simulink model "HardwareM2Eq5"  (R2015a)
settings: configuration reference "SIMULATION_CONFIGURATION" (kept outside this file)
settings Model: DSRTSU_INTERNAL_RTI_VER=400  DSRTSU_INTERNAL_RTI_TYPE=rti1103  SimulationMode=accelerator  CovSFcnEnable=off  Creator=DIT  LastModifiedBy=moritz
settings ConfigSetRef: SourceLocation=Base Workspace

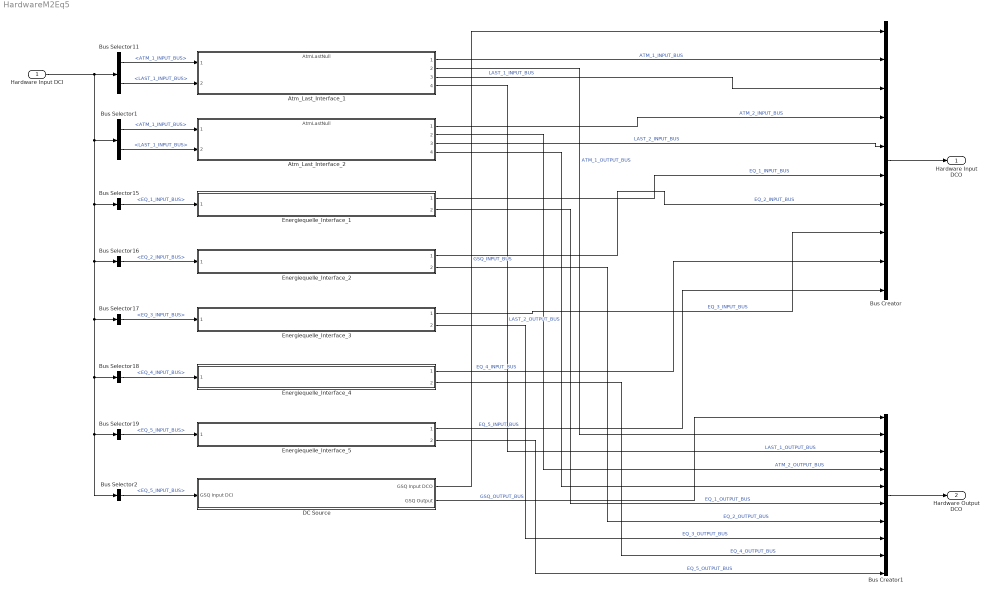
== system HardwareM2Eq5 ==
  Hardware Input DCI : Inport  OutDataTypeStr=Bus: HARDWARE_INPUT_BUS  BusOutputAsStruct=on
  Atm_Last_Interface_1 : ModelReference  ModelNameDialog=AtmLastNull  Variant=on  ModelReferenceVersion=1.18  CopyOfModelName=AtmLastNull  DefaultDataLogging=on
      settings: AttributesFormatString=%<ActiveVariant>
  Atm_Last_Interface_2 : ModelReference  ModelNameDialog=AtmLastNull  Variant=on  ModelReferenceVersion=1.18  CopyOfModelName=AtmLastNull  DefaultDataLogging=on
      settings: AttributesFormatString=%<ActiveVariant>
  Bus Creator : BusCreator  Inputs=10
  Bus Creator1 : BusCreator  Inputs=10  OutDataTypeStr=Bus: HARDWARE_OUTPUT_BUS
  Bus Selector1 : BusSelector  OutputSignals=ATM_1_INPUT_BUS,LAST_1_INPUT_BUS
  Bus Selector11 : BusSelector  OutputSignals=ATM_1_INPUT_BUS,LAST_1_INPUT_BUS
  Bus Selector15 : BusSelector  OutputSignals=EQ_1_INPUT_BUS
  Bus Selector16 : BusSelector  OutputSignals=EQ_2_INPUT_BUS
  Bus Selector17 : BusSelector  OutputSignals=EQ_3_INPUT_BUS
  Bus Selector18 : BusSelector  OutputSignals=EQ_4_INPUT_BUS
  Bus Selector19 : BusSelector  OutputSignals=EQ_5_INPUT_BUS
  Bus Selector2 : BusSelector  OutputSignals=EQ_5_INPUT_BUS
  DC Source : Subsystem
  Energiequelle_Interface_1 : ModelReference  ModelNameDialog=EqReal  Variant=on  ModelReferenceVersion=1.24  DefaultDataLogging=on
      settings: AttributesFormatString=%<ActiveVariant>
  Energiequelle_Interface_2 : ModelReference  ModelNameDialog=EqVirtuellNull.mdl  Variant=on  ModelReferenceVersion=1.24  CopyOfModelName=EqVirtuellNull.mdl  DefaultDataLogging=on
      settings: AttributesFormatString=%<ActiveVariant>
  Energiequelle_Interface_3 : ModelReference  ModelNameDialog=EqVirtuellNull.mdl  Variant=on  ModelReferenceVersion=1.24  CopyOfModelName=EqVirtuellNull.mdl  DefaultDataLogging=on
      settings: AttributesFormatString=%<ActiveVariant>
  Energiequelle_Interface_4 : ModelReference  ModelNameDialog=EqVirtuellNull.mdl  Variant=on  ModelReferenceVersion=1.24  CopyOfModelName=EqVirtuellNull.mdl  DefaultDataLogging=on
      settings: AttributesFormatString=%<ActiveVariant>
  Energiequelle_Interface_5 : ModelReference  ModelNameDialog=EqVirtuellSimple.mdl  Variant=on  ModelReferenceVersion=1.24  DefaultDataLogging=on
      settings: AttributesFormatString=%<ActiveVariant>
  Hardware Input DCO : Outport  OutDataTypeStr=Bus: HARDWARE_INPUT_BUS  BusOutputAsStruct=on
  Hardware Output DCO : Outport  Port=2  OutDataTypeStr=Bus: HARDWARE_OUTPUT_BUS  BusOutputAsStruct=on
  wires:
  Bus Selector11/1 -> Atm_Last_Interface_1/1  "<ATM_1_INPUT_BUS>"
  Bus Selector11/2 -> Atm_Last_Interface_1/2  "<LAST_1_INPUT_BUS>"
  Bus Selector1/1 -> Atm_Last_Interface_2/1  "<ATM_1_INPUT_BUS>"
  Bus Selector1/2 -> Atm_Last_Interface_2/2  "<LAST_1_INPUT_BUS>"
  Bus Selector15/1 -> Energiequelle_Interface_1/1  "<EQ_1_INPUT_BUS>"
  Bus Selector16/1 -> Energiequelle_Interface_2/1  "<EQ_2_INPUT_BUS>"
  Bus Selector17/1 -> Energiequelle_Interface_3/1  "<EQ_3_INPUT_BUS>"
  Bus Selector18/1 -> Energiequelle_Interface_4/1  "<EQ_4_INPUT_BUS>"
  Bus Selector19/1 -> Energiequelle_Interface_5/1  "<EQ_5_INPUT_BUS>"
  Atm_Last_Interface_1/1 -> Bus Creator/2  "ATM_1_INPUT_BUS"
  Atm_Last_Interface_1/3 -> Bus Creator/3  "LAST_1_INPUT_BUS"
  Atm_Last_Interface_1/2 -> Bus Creator1/2  "ATM_1_OUTPUT_BUS"
  Atm_Last_Interface_1/4 -> Bus Creator1/3  "LAST_1_OUTPUT_BUS"
  Atm_Last_Interface_2/1 -> Bus Creator/4  "ATM_2_INPUT_BUS"
  Atm_Last_Interface_2/2 -> Bus Creator1/4  "ATM_2_OUTPUT_BUS"
  Atm_Last_Interface_2/3 -> Bus Creator/5  "LAST_2_INPUT_BUS"
  Atm_Last_Interface_2/4 -> Bus Creator1/5  "LAST_2_OUTPUT_BUS"
  Energiequelle_Interface_1/1 -> Bus Creator/6  "EQ_1_INPUT_BUS"
  Energiequelle_Interface_1/2 -> Bus Creator1/6  "EQ_1_OUTPUT_BUS"
  Energiequelle_Interface_5/2 -> Bus Creator1/10  "EQ_5_OUTPUT_BUS"
  Energiequelle_Interface_5/1 -> Bus Creator/10  "EQ_5_INPUT_BUS"
  Energiequelle_Interface_4/2 -> Bus Creator1/9  "EQ_4_OUTPUT_BUS"
  Energiequelle_Interface_4/1 -> Bus Creator/9  "EQ_4_INPUT_BUS"
  Energiequelle_Interface_3/2 -> Bus Creator1/8  "EQ_3_OUTPUT_BUS"
  Energiequelle_Interface_3/1 -> Bus Creator/8  "EQ_3_INPUT_BUS"
  Energiequelle_Interface_2/2 -> Bus Creator1/7  "EQ_2_OUTPUT_BUS"
  Energiequelle_Interface_2/1 -> Bus Creator/7  "EQ_2_INPUT_BUS"
  Bus Creator/1 -> Hardware Input DCO/1
  Bus Creator1/1 -> Hardware Output DCO/1
  DC Source/1(GSQ Input DCO) -> Bus Creator/1  "GSQ_INPUT_BUS"
  DC Source/2(GSQ Output) -> Bus Creator1/1  "GSQ_OUTPUT_BUS"
  Hardware Input DCI/1 -> Bus Selector2/1, Bus Selector19/1, Bus Selector18/1, Bus Selector17/1, Bus Selector16/1, Bus Selector15/1, Bus Selector1/1, Bus Selector11/1
  Bus Selector2/1 -> DC Source/1(GSQ Input DCI)  "<EQ_5_INPUT_BUS>"

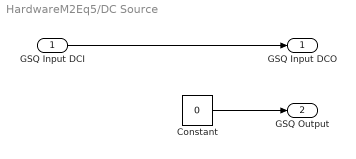
== system HardwareM2Eq5/DC Source ==
  GSQ Input DCI : Inport
  Constant : Constant  Value=0  OutDataTypeStr=Bus: GSQ_OUTPUT_BUS
  GSQ Input DCO : Outport  OutDataTypeStr=Bus: GSQ_INPUT_BUS
  GSQ Output : Outport  Port=2  OutDataTypeStr=Bus: GSQ_OUTPUT_BUS
  wires:
  GSQ Input DCI/1 -> GSQ Input DCO/1
  Constant/1 -> GSQ Output/1
